simulink model "MATE_IEEE123Node"  (R2024b)
settings: Solver=FixedStepDiscrete  StartTime=0.0  StopTime=1  FixedStep=Ts  RelTol=1e-3
PostLoadFcn:
  | Ts=50e-6;init_IEEE123Node;
InitFcn:
  | Ts=50e-6;init_IEEE123Node;
undefined symbols (not defined in the file): ft2km, loadcoeff, MATE, MATERT, Pa1, Pa13, Pa14, Pa17, Pa18, Pa22, Pa24, Pa25, Pa29, Pa31, Pa32, Pa33, Pa34, Pa35, Pa37, Pa38, Pa39, Pa44, Pa46, Pa48, Pa50, Pa51, Pa52, Pa53, Pa57, Pa59, Pa6, Pa61, Pa67, Pa7, Pa70, Pa73, Pa8, Pa81, Pa82, Pa83, Pa84, Pa85, Pa9, Pb10, Pb15, Pb2, Pb30, Pb33, Pb34, Pb35, Pb41, Pb42, Pb43, Pb47, Pb48, Pb57, Pb58, Pb60, Pb65, Pb66 ... (+124)
libraries: simetranss x259, ee_lib x93, fl_lib x67, nesl_utility x67, simetran x2
(part 2 of 4)

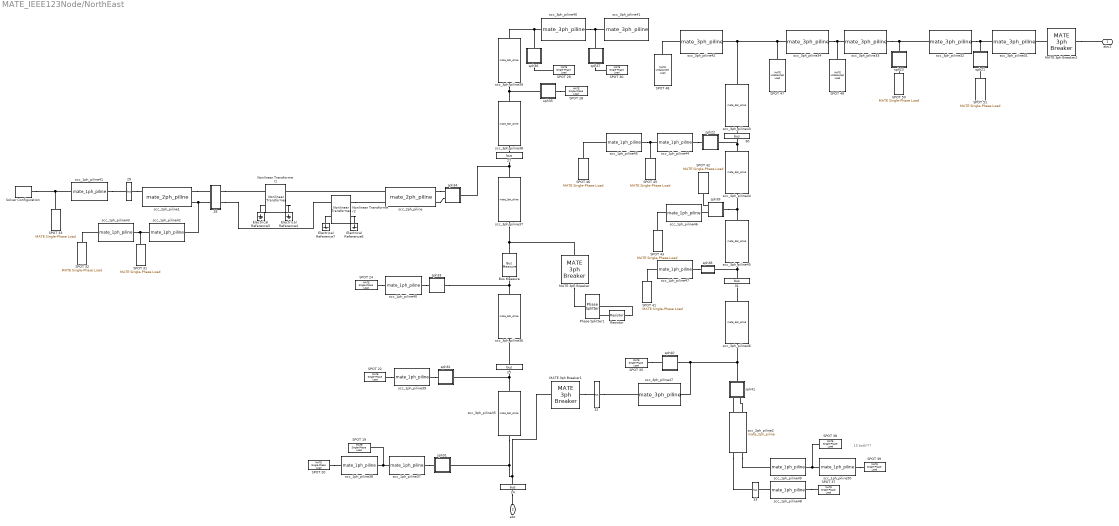
== system MATE_IEEE123Node/NorthEast ==
  note: 15 both???
  24 : simetranss/Measure/bus  bn=18
      settings: AttributesFormatString=Bus %<bn>
  25 : simetranss/Measure/bus  bn=21
      settings: AttributesFormatString=Bus %<bn>
  27 : simetranss/Measure/bus  bn=25
      settings: AttributesFormatString=Bus %<bn>
  28 : Subsystem  AncestorBlock=simetran/5  mask(Simscape Electrical Bus Numbering){bn=26}
      mask prompts: bn "Bus number"
      mask help: This block is a simple passthrough
      settings: AttributesFormatString=Bus %<bn>
  29 : simetranss/Measure/bus  bn=27
      settings: AttributesFormatString=Bus %<bn>
  30 : simetranss/Measure/bus  bn=44
      settings: AttributesFormatString=Bus %<bn>
  31 : simetranss/Measure/bus  bn=40
      settings: AttributesFormatString=Bus %<bn>
  32 : simetranss/Measure/bus  bn=135
      settings: AttributesFormatString=Bus %<bn>
  33 : simetranss/Measure/bus  bn=36
      settings: AttributesFormatString=Bus %<bn>
  Bus Measure : simetranss/Measure/Bus Measure  VoltageMeasurement=phase-to-ground  SetLabelV=on  LabelV=Vabc_B1ssc  Vpu=off  VpuLL=off  CurrentMeasurement=yes  SetLabelI=on  LabelI=Iabc_B1ssc  Ipu=off  Pbase=100e6  Vbase=500e3  bnumber=23  dis=off
  Electrical Reference{4..7} (4 alike) : fl_lib/Electrical/Electrical Elements/Electrical Reference
  MATE 3ph Breaker : simetranss/Switches/MATE 3ph Breaker  InitialState=open  SwitchA=off  SwitchB=on  SwitchC=on  SwitchTimes=[0.5 0.5+3/60]  External=off  BreakerResistance=0.01  Roff=1e6  SnubberResistance=1e6  SnubberCapacitance=inf
  MATE 3ph Breaker1 : simetranss/Switches/MATE 3ph Breaker  InitialState=closed  SwitchA=off  SwitchB=off  SwitchC=off  SwitchTimes="[1/60  5/60]"  External=off  BreakerResistance=0.01  Roff=1e6  SnubberResistance=1e6  SnubberCapacitance=inf
  MATE 3ph Breaker2 : simetranss/Switches/MATE 3ph Breaker  InitialState=closed  SwitchA=off  SwitchB=off  SwitchC=off  SwitchTimes="[1/60  5/60]"  External=off  BreakerResistance=0.01  Roff=1e6  SnubberResistance=1e6  SnubberCapacitance=inf
  Nonlinear Transformer1 : ee_lib/Passive/Transformers/Nonlinear Transformer  Nw=1  Nw2=1  winding_param_option=2  Req=0.01 Ohm  Leq=0.0001 H  R_1=0.087552 Ohm  L_1=0.011426 H  R_2=0.27563 Ohm  L_2=0.035971 H  averaging_period=0 s  R_m=50000 Ohm  parameterization_option=1  H_data=[0, 200, 400, 600, 800, 1000] A/m  B_data=[0, .81, 1.25, 1.42, 1.48, 1.49] T  length_effective=0.2 m  area_effective=2e-4 m^2  L=1 H  L_sat=1e-2 H  current_data=[0, .4, .8, 1.2, 1.6, 2] A  magnetic_flux_data=[0, .161, .25, .284, .295, .299] .* 1e-3 Wb  magnetic_flux_sat=1.6e-04 Wb  dBdH0=0.005 T*m/A  B1=1.49 T  H1=1000 A/m  c=0.1  K=200 A/m  alpha=1e-4  interpolation_option=1  Leq_i0=0 A  L1_i0=0 A  L2_i0=0 A  x0_option=1  i_L0=0 A  phi0=0 Wb  B0=0 T  H0=0 A/m  Leq_g=1e-9 1/Ohm  L1_g=1e-9 1/Ohm  L2_g=1e-9 1/Ohm
      settings: InternalSimscapePortConfiguration="{\"Bottom\":[],\"Left\":[{\"id\":\"p1\",\"label\":\"1+\",\"type\":\"foundation.electrical.electrical\"},{\"id\":\"n1\",\"label\":\"1-\",\"type\":\"foundation.electrical.electrical\"}],\"Right\":[{\"id\":\"p2\",\"label\":\"2+\",\"type\":\"foundation.electrical.electrical\"},{\"id\":\"n2\",\"label\":\"2-\",\"type\":\"foundation.electrical.electrical\"}],\"Top\":[]}"
  Nonlinear Transformer2 : ee_lib/Passive/Transformers/Nonlinear Transformer  Nw=1  Nw2=1  winding_param_option=2  Req=0.01 Ohm  Leq=0.0001 H  R_1=0.087552 Ohm  L_1=0.011426 H  R_2=0.27563 Ohm  L_2=0.035971 H  averaging_period=0 s  R_m=50000 Ohm  parameterization_option=1  H_data=[0, 200, 400, 600, 800, 1000] A/m  B_data=[0, .81, 1.25, 1.42, 1.48, 1.49] T  length_effective=0.2 m  area_effective=2e-4 m^2  L=1 H  L_sat=1e-2 H  current_data=[0, .4, .8, 1.2, 1.6, 2] A  magnetic_flux_data=[0, .161, .25, .284, .295, .299] .* 1e-3 Wb  magnetic_flux_sat=1.6e-04 Wb  dBdH0=0.005 T*m/A  B1=1.49 T  H1=1000 A/m  c=0.1  K=200 A/m  alpha=1e-4  interpolation_option=1  Leq_i0=0 A  L1_i0=0 A  L2_i0=0 A  x0_option=1  i_L0=0 A  phi0=0 Wb  B0=0 T  H0=0 A/m  Leq_g=1e-9 1/Ohm  L1_g=1e-9 1/Ohm  L2_g=1e-9 1/Ohm
      settings: InternalSimscapePortConfiguration="{\"Bottom\":[],\"Left\":[{\"id\":\"p1\",\"label\":\"1+\",\"type\":\"foundation.electrical.electrical\"},{\"id\":\"n1\",\"label\":\"1-\",\"type\":\"foundation.electrical.electrical\"}],\"Right\":[{\"id\":\"p2\",\"label\":\"2+\",\"type\":\"foundation.electrical.electrical\"},{\"id\":\"n2\",\"label\":\"2-\",\"type\":\"foundation.electrical.electrical\"}],\"Top\":[]}"
  Phase Splitter1 : ee_lib/Connectors & References/Phase Splitter
  Resistor : ee_lib/Passive/Resistor  R=0.001 Ohm  enable_R_tol=ee.enum.toleranceApplication.none  R_tol=5  tol_distribution=ee.enum.toleranceDistribution.uniform  nSigma=4  enable_operating_limits=ee.enum.enable.no  operating_limit_action=ee.enum.passive.reportOpLim.warn  power_rating=1 W  max_working_voltage=100 V  noise_mode=ee.enum.sources.noise.Disabled  Tdevice=25 degC  sample_time=1e-3 s  repeatability=ee.enum.ic.repeatability.notRepeatable  user_seed=0  auto_seed=2080827355  fault_action=simscape.enum.assert.action.none  t_fault=1 s  power_derating_T1=70 degC  power_derating_T2=155 degC  operating_temperature_range_vec=[-50, 150] degC  alpha=3.93e-3 1/K  Tmeas=25 degC  thermal_mass=100 J/K  temperature_specify=off  temperature_priority=High  temperature=298.15 K  temperature_nominal_specify=off  temperature_nominal_value=1  temperature_nominal_unit=K
  SPOT 19 : simetranss/Passive/MATE Single-Phase Load  Vabc=VsubL/sqrt(3)  Fn=60  typ=Series RL  Pabc=Pa13*loadcoeff  QLabc=Qa13*loadcoeff  QCabc="[190  ]*1e3"
  SPOT 20 : simetranss/Passive/MATE Single-Phase Load  Vabc=VsubL/sqrt(3)  Fn=60  typ=Series RL  Pabc=Pa14*loadcoeff  QLabc=Qa14*loadcoeff  QCabc="[190  ]*1e3"
  SPOT 22 : simetranss/Passive/MATE Single-Phase Load  Vabc=VsubL/sqrt(3)  Fn=60  typ=Series RL  Pabc=Pb15*loadcoeff  QLabc=Qb15*loadcoeff  QCabc="[190  ]*1e3"
  SPOT 24 : simetranss/Passive/MATE Single-Phase Load  Vabc=VsubL/sqrt(3)  Fn=60  typ=Series RL  Pabc=Pc16*loadcoeff  QLabc=Qc16*loadcoeff  QCabc="[190  ]*1e3"
  SPOT 28 : simetranss/Passive/MATE Single-Phase Load  Vabc=VsubL/sqrt(3)  Fn=60  typ=Series RL  Pabc=Pa17*loadcoeff  QLabc=Qa17*loadcoeff  QCabc="[190  ]*1e3"
  SPOT 29 : simetranss/Passive/MATE Single-Phase Load  Vabc=VsubL/sqrt(3)  Fn=60  typ=Series RL  Pabc=Pa18*loadcoeff  QLabc=Qa18*loadcoeff  QCabc="[190  ]*1e3"
  SPOT 30 : simetranss/Passive/MATE Single-Phase Load  Vabc=VsubL/sqrt(3)  Fn=60  typ=Series RL  Pabc=Pc19*loadcoeff  QLabc=Qc19*loadcoeff  QCabc="[190  ]*1e3"
  SPOT 31 : simetranss/Passive/MATE Single-Phase Load  Vabc=VsubL/sqrt(3)  Fn=60  typ=Series RL  Pabc=Pc20*loadcoeff  QLabc=Qc20*loadcoeff  QCabc="[190  ]*1e3"
  SPOT 32 : simetranss/Passive/MATE Single-Phase Load  Vabc=VsubL/sqrt(3)  Fn=60  typ=Series RL  Pabc=Pc21*loadcoeff  QLabc=Qc21*loadcoeff  QCabc="[190  ]*1e3"
  SPOT 33 : simetranss/Passive/MATE Single-Phase Load  Vabc=VsubL/sqrt(3)  Fn=60  typ=Series RL  Pabc=Pa22*loadcoeff  QLabc=Qa22*loadcoeff  QCabc="[190  ]*1e3"
  SPOT 35 : simetranss/Passive/MATE Single-Phase Load  Vabc=VsubL/sqrt(3)  Fn=60  typ=Series RL  Pabc=Pa24*loadcoeff  QLabc=Qa24*loadcoeff  QCabc="[190  ]*1e3"
  SPOT 37 : simetranss/Passive/MATE Single-Phase Load  Vabc=VsubL/sqrt(3)  Fn=60  typ=Series RL  Pabc=Pa25*loadcoeff  QLabc=Qa25*loadcoeff  QCabc="[190  ]*1e3"
  SPOT 38 : simetranss/Passive/MATE Single-Phase Load  Vabc=VsubL/sqrt(3)  Fn=60  typ=Series RL  Pabc=Pb15*loadcoeff  QLabc=Qb15*loadcoeff  QCabc="[190  ]*1e3"
  SPOT 39 : simetranss/Passive/MATE Single-Phase Load  Vabc=VsubL/sqrt(3)  Fn=60  typ=Series RL  Pabc=Pb15*loadcoeff  QLabc=Qb15*loadcoeff  QCabc="[190  ]*1e3"
  SPOT 41 : simetranss/Passive/MATE Single-Phase Load  Vabc=VsubL/sqrt(3)  Fn=60  typ=Series RL  Pabc=Pc28*loadcoeff  QLabc=Qc28*loadcoeff  QCabc="[190  ]*1e3"
  SPOT 42 : simetranss/Passive/MATE Single-Phase Load  Vabc=VsubL/sqrt(3)  Fn=60  typ=Series RL  Pabc=Pa29*loadcoeff  QLabc=Qa29*loadcoeff  QCabc="[190  ]*1e3"
  SPOT 43 : simetranss/Passive/MATE Single-Phase Load  Vabc=VsubL/sqrt(3)  Fn=60  typ=Series RL  Pabc=Pb30*loadcoeff  QLabc=Qb30*loadcoeff  QCabc="[190  ]*1e3"
  SPOT 45 : simetranss/Passive/MATE Single-Phase Load  Vabc=VsubL/sqrt(3)  Fn=60  typ=Series RL  Pabc=Pa31*loadcoeff  QLabc=Qa31*loadcoeff  QCabc="[190  ]*1e3"
  SPOT 46 : simetranss/Passive/MATE Single-Phase Load  Vabc=VsubL/sqrt(3)  Fn=60  typ=Series RL  Pabc=Pa32*loadcoeff  QLabc=Qa32*loadcoeff  QCabc="[190  ]*1e3"
  SPOT 47 : simetranss/Passive/MATE Unbalanced Load  Vabc=[ 0.993926 1.02168 0.995885]*277.128  Fn=60  typ=Series RL  Pabc=[Pa33*loadcoeff Pb33*loadcoeff Pc33*loadcoeff]  QLabc=[Qa33*loadcoeff Qb33*loadcoeff Qc33*loadcoeff]  QCabc="[190  60  212]*1e3"
  SPOT 48 : simetranss/Passive/MATE Unbalanced Load  Vabc=[ 0.993926 1.02168 0.995885]*277.128  Fn=60  typ=Series RL  Pabc=[Pa34*loadcoeff Pb34*loadcoeff Pc34*loadcoeff]  QLabc=[Qa34*loadcoeff Qb34*loadcoeff Qc34*loadcoeff]  QCabc="[190  60  212]*1e3"
  SPOT 49 : simetranss/Passive/MATE Unbalanced Load  Vabc=[ 0.993926 1.02168 0.995885]*277.128  Fn=60  typ=Series RL  Pabc=[Pa35*loadcoeff Pb35*loadcoeff Pc35*loadcoeff]  QLabc=[Qa35*loadcoeff Qb35*loadcoeff Qc35*loadcoeff]  QCabc="[190  60  212]*1e3"
  SPOT 50 : simetranss/Passive/MATE Single-Phase Load  Vabc=VsubL/sqrt(3)  Fn=60  typ=Series RL  Pabc=Pc36*loadcoeff  QLabc=Qc36*loadcoeff  QCabc="[190  ]*1e3"
  SPOT 51 : simetranss/Passive/MATE Single-Phase Load  Vabc=VsubL/sqrt(3)  Fn=60  typ=Series RL  Pabc=Pa37*loadcoeff  QLabc=Qa37*loadcoeff  QCabc="[190  ]*1e3"
  Solver Configuration : nesl_utility/Solver Configuration  PhysicalDomain=network_engine_domain  SubClassName=solver  LeftPortType=input  RightPortType=generic  Tones=[]  Harmonics=[]  SimulateNoise=off  Profile=off  UseLocalSampling=off  EnableSwitchedLinearOptims=on  FrequencyDomain=off  UseCCode=off  RelTol=0.001  AbsTol=0.001  MinStep=1e-09  ToWorkspace=off  RevertToSquareIcSolve=off  NumHomotopyIterations=100  PhasorMode=off  PhasorModeNumHarmonics=1  ConsistencySolver=NEWTON_XTOL_AFTER_FTOL  IndexReductionMethod=None  DoDC=off  ResidualTolerance=1e-09  ConsistencyTolSource=GLOBAL  ConsistencyAbsTol=0.001  ConsistencyRelTol=0.001  ConsistencyTolFactor=0.1  UseLocalSolver=on  LocalSolverChoice=NE_PARTITIONING_ADVANCER  ResolveIndetEquations=off  FunctionEvalNumThread=1  LocalSolverSampleTime=Ts  DoFixedCost=on  MaxNonlinIter=1  MaxModeIter=2  ComputeImpulses=off  ImpulseIterations=2  LinearAlgebra=auto  LinearAlgebraNumThread=0  EquationFormulation=NE_TIME_EF  DelaysMemoryBudget=1024  AutomaticFiltering=on  FilteringTimeConstant=0.001  PartitionStorageMethod=AS_NEEDED  PartitionMemoryBudget=1024  PartitionMethod=ROBUST  MultibodyUseLocalSolver=off  MultibodyLocalSolverChoice=ODE1  MultibodyLocalSolverSampleTime=0.001
  scc_1ph_piline37 : simetranss/Lines/mate_1ph_piline  FF=60  conf=config 9  lenfeet=250  dmi=off  RR1=0.8  LL1=0.002  CC1=7e-9  lenkm=1
  scc_1ph_piline38 : simetranss/Lines/mate_1ph_piline  FF=60  conf=config 9  lenfeet=325  dmi=off  RR1=0.8  LL1=0.002  CC1=7e-9  lenkm=1
  scc_1ph_piline39 : simetranss/Lines/mate_1ph_piline  FF=60  conf=config 10  lenfeet=525  dmi=off  RR1=0.8  LL1=0.002  CC1=7e-9  lenkm=1
  scc_1ph_piline40 : simetranss/Lines/mate_1ph_piline  FF=60  conf=config 11  lenfeet=550  dmi=off  RR1=0.8  LL1=0.002  CC1=7e-9  lenkm=1
  scc_1ph_piline41 : simetranss/Lines/mate_1ph_piline  FF=60  conf=config 9  lenfeet=500  dmi=off  RR1=0.8  LL1=0.002  CC1=7e-9  lenkm=1
  scc_1ph_piline42 : simetranss/Lines/mate_1ph_piline  FF=60  conf=config 11  lenfeet=225  dmi=off  RR1=0.8  LL1=0.002  CC1=7e-9  lenkm=1
  scc_1ph_piline43 : simetranss/Lines/mate_1ph_piline  FF=60  conf=config 11  lenfeet=300  dmi=off  RR1=0.8  LL1=0.002  CC1=7e-9  lenkm=1
  scc_1ph_piline44 : simetranss/Lines/mate_1ph_piline  FF=60  conf=config 9  lenfeet=200  dmi=off  RR1=0.8  LL1=0.002  CC1=7e-9  lenkm=1
  scc_1ph_piline45 : simetranss/Lines/mate_1ph_piline  FF=60  conf=config 9  lenfeet=300  dmi=off  RR1=0.8  LL1=0.002  CC1=7e-9  lenkm=1
  scc_1ph_piline46 : simetranss/Lines/mate_1ph_piline  FF=60  conf=config 10  lenfeet=500  dmi=off  RR1=0.8  LL1=0.002  CC1=7e-9  lenkm=1
  scc_1ph_piline47 : simetranss/Lines/mate_1ph_piline  FF=60  conf=config 11  lenfeet=325  dmi=off  RR1=0.8  LL1=0.002  CC1=7e-9  lenkm=1
  scc_1ph_piline48 : simetranss/Lines/mate_1ph_piline  FF=60  conf=config 9  lenfeet=300  dmi=off  RR1=0.8  LL1=0.002  CC1=7e-9  lenkm=1
  scc_1ph_piline49 : simetranss/Lines/mate_1ph_piline  FF=60  conf=config 10  lenfeet=250  dmi=off  RR1=0.8  LL1=0.002  CC1=7e-9  lenkm=1
  scc_1ph_piline50 : simetranss/Lines/mate_1ph_piline  FF=60  conf=config 10  lenfeet=325  dmi=off  RR1=0.8  LL1=0.002  CC1=7e-9  lenkm=1
  scc_2ph_piline : simetranss/Lines/mate_2ph_piline  FF=60  conf=config 7  lenfeet=350  dmi=off  RR22=[1 0; 0 1]  LL22=[1 0; 0 1]  CC22=[1 0; 0 1]  lenkm=1
  scc_2ph_piline1 : simetranss/Lines/mate_2ph_piline  FF=60  conf=config 7  lenfeet=275  dmi=off  RR22=[1 0; 0 1]  LL22=[1 0; 0 1]  CC22=[1 0; 0 1]  lenkm=1
  scc_2ph_piline2 : simetranss/Lines/mate_2ph_piline  FF=60  conf=config 8  lenfeet=650  dmi=off  RR22=[1 0; 0 1]  LL22=[1 0; 0 1]  CC22=[1 0; 0 1]  lenkm=1
  scc_3ph_piline31 : simetranss/Lines/mate_3ph_piline  FF=60  conf=config 5  lenfeet=500  dmi=off  RR33=[1 0 0;0 1 0; 0 0 1]  LL33=[1 0 0;0 1 0; 0 0 1]  CC33=[1 0 0;0 1 0; 0 0 1]  lenkm=1
  scc_3ph_piline32 : simetranss/Lines/mate_3ph_piline  FF=60  conf=config 4  lenfeet=250  dmi=off  RR33=[1 0 0;0 1 0; 0 0 1]  LL33=[1 0 0;0 1 0; 0 0 1]  CC33=[1 0 0;0 1 0; 0 0 1]  lenkm=1
  scc_3ph_piline33 : simetranss/Lines/mate_3ph_piline  FF=60  conf=config 4  lenfeet=250  dmi=off  RR33=[1 0 0;0 1 0; 0 0 1]  LL33=[1 0 0;0 1 0; 0 0 1]  CC33=[1 0 0;0 1 0; 0 0 1]  lenkm=1
  scc_3ph_piline34 : simetranss/Lines/mate_3ph_piline  FF=60  conf=config 4  lenfeet=250  dmi=off  RR33=[1 0 0;0 1 0; 0 0 1]  LL33=[1 0 0;0 1 0; 0 0 1]  CC33=[1 0 0;0 1 0; 0 0 1]  lenkm=1
  scc_3ph_piline35 : simetranss/Lines/mate_3ph_piline  FF=60  conf=config 2  lenfeet=300  dmi=off  RR33=[1 0 0;0 1 0; 0 0 1]  LL33=[1 0 0;0 1 0; 0 0 1]  CC33=[1 0 0;0 1 0; 0 0 1]  lenkm=1
  scc_3ph_piline36 : simetranss/Lines/mate_3ph_piline  FF=60  conf=config 2  lenfeet=250  dmi=off  RR33=[1 0 0;0 1 0; 0 0 1]  LL33=[1 0 0;0 1 0; 0 0 1]  CC33=[1 0 0;0 1 0; 0 0 1]  lenkm=1
  scc_3ph_piline37 : simetranss/Lines/mate_3ph_piline  FF=60  conf=config 2  lenfeet=275  dmi=off  RR33=[1 0 0;0 1 0; 0 0 1]  LL33=[1 0 0;0 1 0; 0 0 1]  CC33=[1 0 0;0 1 0; 0 0 1]  lenkm=1
  scc_3ph_piline38 : simetranss/Lines/mate_3ph_piline  FF=60  conf=config 2  lenfeet=200  dmi=off  RR33=[1 0 0;0 1 0; 0 0 1]  LL33=[1 0 0;0 1 0; 0 0 1]  CC33=[1 0 0;0 1 0; 0 0 1]  lenkm=1
  scc_3ph_piline39 : simetranss/Lines/mate_3ph_piline  FF=60  conf=config 2  lenfeet=300  dmi=off  RR33=[1 0 0;0 1 0; 0 0 1]  LL33=[1 0 0;0 1 0; 0 0 1]  CC33=[1 0 0;0 1 0; 0 0 1]  lenkm=1
  scc_3ph_piline40 : simetranss/Lines/mate_3ph_piline  FF=60  conf=config 2  lenfeet=350  dmi=off  RR33=[1 0 0;0 1 0; 0 0 1]  LL33=[1 0 0;0 1 0; 0 0 1]  CC33=[1 0 0;0 1 0; 0 0 1]  lenkm=1
  scc_3ph_piline41 : simetranss/Lines/mate_3ph_piline  FF=60  conf=config 2  lenfeet=200  dmi=off  RR33=[1 0 0;0 1 0; 0 0 1]  LL33=[1 0 0;0 1 0; 0 0 1]  CC33=[1 0 0;0 1 0; 0 0 1]  lenkm=1
  scc_3ph_piline42 : simetranss/Lines/mate_3ph_piline  FF=60  conf=config 4  lenfeet=150  dmi=off  RR33=[1 0 0;0 1 0; 0 0 1]  LL33=[1 0 0;0 1 0; 0 0 1]  CC33=[1 0 0;0 1 0; 0 0 1]  lenkm=1
  scc_3ph_piline43 : simetranss/Lines/mate_3ph_piline  FF=60  conf=config 1  lenfeet=250  dmi=off  RR33=[1 0 0;0 1 0; 0 0 1]  LL33=[1 0 0;0 1 0; 0 0 1]  CC33=[1 0 0;0 1 0; 0 0 1]  lenkm=1
  scc_3ph_piline44 : simetranss/Lines/mate_3ph_piline  FF=60  conf=config 1  lenfeet=200  dmi=off  RR33=[1 0 0;0 1 0; 0 0 1]  LL33=[1 0 0;0 1 0; 0 0 1]  CC33=[1 0 0;0 1 0; 0 0 1]  lenkm=1
  scc_3ph_piline45 : simetranss/Lines/mate_3ph_piline  FF=60  conf=config 1  lenfeet=250  dmi=off  RR33=[1 0 0;0 1 0; 0 0 1]  LL33=[1 0 0;0 1 0; 0 0 1]  CC33=[1 0 0;0 1 0; 0 0 1]  lenkm=1
  scc_3ph_piline46 : simetranss/Lines/mate_3ph_piline  FF=60  conf=config 1  lenfeet=250  dmi=off  RR33=[1 0 0;0 1 0; 0 0 1]  LL33=[1 0 0;0 1 0; 0 0 1]  CC33=[1 0 0;0 1 0; 0 0 1]  lenkm=1
  scc_3ph_piline47 : simetranss/Lines/mate_3ph_piline  FF=60  conf=config 4  lenfeet=375  dmi=off  RR33=[1 0 0;0 1 0; 0 0 1]  LL33=[1 0 0;0 1 0; 0 0 1]  CC33=[1 0 0;0 1 0; 0 0 1]  lenkm=1
  sph21 : Subsystem
  sph22 : Subsystem
  sph23 : Subsystem
  sph31 : Subsystem
  sph32 : Subsystem
  sph33 : Subsystem
  sph34 : Subsystem
  sph35 : Subsystem
  sph36 : Subsystem
  sph37 : Subsystem
  sph38 : Subsystem
  sph39 : Subsystem
  sph40 : Subsystem
  sph41 : Subsystem
  abc2 : PMIOPort  Side=Right
  abc : PMIOPort  Port=2  Side=Left
  connections:
  scc_3ph_piline34/LConn1 -- SPOT 47/LConn1 -- scc_3ph_piline42/RConn1 -- scc_3ph_piline43/LConn1
  27/LConn1 -- scc_3ph_piline37/LConn1 -- sph34/LConn1
  scc_3ph_piline32/RConn1 -- scc_3ph_piline31/LConn1 -- sph21/LConn1
  scc_3ph_piline46/RConn1 -- scc_3ph_piline47/LConn1 -- sph40/LConn1 -- sph41/LConn1
  scc_3ph_piline34/RConn1 -- scc_3ph_piline33/LConn1 -- SPOT 49/LConn1
  scc_3ph_piline39/LConn1 -- sph36/LConn1 -- scc_3ph_piline40/RConn1
  scc_1ph_piline46/RConn1 -- SPOT 43/LConn1
  scc_1ph_piline43/LConn1 -- SPOT 32/LConn1
  scc_3ph_piline37/RConn1 -- Bus Measure/LConn1 -- MATE 3ph Breaker/LConn1
  scc_2ph_piline2/RConn2 -- scc_1ph_piline49/RConn1
  SPOT 41/LConn1 -- scc_1ph_piline47/RConn1
  scc_1ph_piline39/LConn1 -- sph32/RConn1
  30/RConn1 -- scc_3ph_piline43/RConn1
  28/RConn2 -- Nonlinear Transformer2/LConn1
  scc_3ph_piline35/LConn1 -- 25/LConn1 -- sph32/LConn1
  scc_2ph_piline2/LConn1 -- sph41/RConn1
  sph37/RConn1 -- SPOT 30/LConn1
  sph39/RConn2 -- scc_1ph_piline46/LConn1
  31/RConn1 -- scc_3ph_piline45/RConn1 -- sph38/LConn1
  scc_3ph_piline44/LConn1 -- sph22/LConn1 -- 30/LConn1
  scc_3ph_piline33/RConn1 -- scc_3ph_piline32/LConn1 -- sph23/LConn1
  SPOT 51/LConn1 -- sph21/RConn1
  scc_1ph_piline48/LConn1 -- SPOT 37/LConn1
  scc_3ph_piline39/RConn1 -- scc_3ph_piline38/LConn1 -- sph35/LConn1
  MATE 3ph Breaker1/LConn1 -- 32/LConn1
  25/RConn1 -- scc_3ph_piline36/RConn1
  scc_3ph_piline46/LConn1 -- 31/LConn1
  Nonlinear Transformer2/LConn2 -- Electrical Reference7/LConn1
  SPOT 22/LConn1 -- scc_1ph_piline39/RConn1
  scc_1ph_piline49/LConn1 -- SPOT 38/LConn1 -- scc_1ph_piline50/RConn1
  sph39/RConn1 -- SPOT 42/LConn1
  scc_2ph_piline1/RConn2 -- scc_1ph_piline42/RConn1 -- 28/LConn2
  28/RConn1 -- Nonlinear Transformer1/LConn1
  scc_2ph_piline2/RConn1 -- 33/LConn1
  sph35/RConn1 -- SPOT 28/LConn1
  Nonlinear Transformer1/LConn2 -- Electrical Reference5/LConn1
  scc_1ph_piline40/LConn1 -- sph33/RConn1
  scc_1ph_piline44/LConn1 -- sph22/RConn1
  scc_1ph_piline47/LConn1 -- sph38/RConn1
  SPOT 20/LConn1 -- scc_1ph_piline38/RConn1
  scc_1ph_piline41/RConn1 -- 29/RConn1
  scc_1ph_piline37/LConn1 -- sph31/RConn1
  MATE 3ph Breaker2/RConn1 -- abc2/RConn1
  scc_1ph_piline38/LConn1 -- SPOT 19/LConn1 -- scc_1ph_piline37/RConn1
  SPOT 50/LConn1 -- sph23/RConn1
  32/RConn1 -- scc_3ph_piline47/RConn1
  MATE 3ph Breaker2/LConn1 -- scc_3ph_piline31/RConn1
  scc_3ph_piline40/LConn1 -- sph37/LConn1 -- scc_3ph_piline41/RConn1
  scc_2ph_piline2/LConn2 -- sph41/RConn2
  scc_1ph_piline48/RConn1 -- 33/RConn1
  scc_2ph_piline1/RConn1 -- 28/LConn1
  scc_3ph_piline44/RConn1 -- sph39/LConn1 -- scc_3ph_piline45/LConn1
  scc_1ph_piline43/RConn1 -- SPOT 31/LConn1 -- scc_1ph_piline42/LConn1
  SPOT 46/LConn1 -- scc_1ph_piline45/RConn1
  SPOT 24/LConn1 -- scc_1ph_piline40/RConn1
  scc_3ph_piline35/RConn1 -- sph31/LConn1 -- MATE 3ph Breaker1/RConn1 -- 24/RConn1
  Nonlinear Transformer2/RConn2 -- Electrical Reference6/LConn1
  sph36/RConn1 -- SPOT 29/LConn1
  scc_3ph_piline38/RConn1 -- 27/RConn1
  scc_1ph_piline45/LConn1 -- SPOT 45/LConn1 -- scc_1ph_piline44/RConn1
  29/LConn1 -- scc_2ph_piline1/LConn1
  scc_2ph_piline/RConn2 -- sph34/RConn2
  Nonlinear Transformer1/RConn2 -- Electrical Reference4/LConn1
  SPOT 33/LConn1 -- Solver Configuration/RConn1 -- scc_1ph_piline41/LConn1
  scc_1ph_piline50/LConn1 -- SPOT 39/LConn1
  SPOT 35/LConn1 -- sph40/RConn1
  scc_2ph_piline/LConn1 -- Nonlinear Transformer1/RConn1
  scc_2ph_piline/RConn1 -- sph34/RConn1
  Nonlinear Transformer2/RConn1 -- scc_2ph_piline/LConn2
  24/LConn1 -- abc/RConn1
  sph33/LConn1 -- Bus Measure/RConn1 -- scc_3ph_piline36/LConn1
  scc_3ph_piline42/LConn1 -- SPOT 48/LConn1
  MATE 3ph Breaker/RConn1 -- Phase Splitter1/LConn1
  Resistor/LConn1 -- Phase Splitter1/RConn3
  Resistor/RConn1 -- Phase Splitter1/RConn2

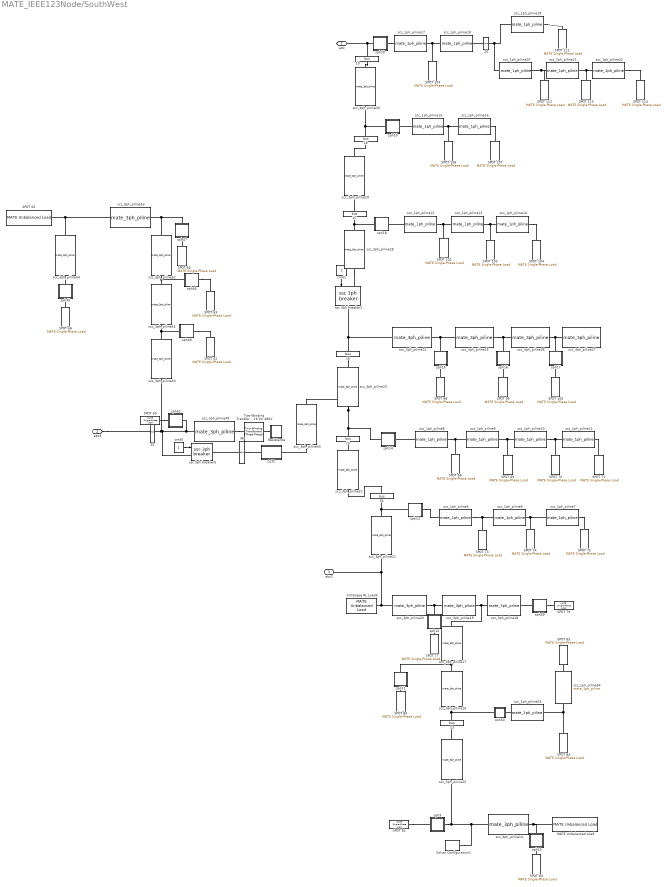
== system MATE_IEEE123Node/SouthWest ==
  13 : simetranss/Measure/bus  bn=61
      settings: AttributesFormatString=Bus %<bn>
  14 : simetranss/Measure/bus  bn=72
      settings: AttributesFormatString=Bus %<bn>
  15 : simetranss/Measure/bus  bn=67
      settings: AttributesFormatString=Bus %<bn>
  16 : simetranss/Measure/bus  bn=97
      settings: AttributesFormatString=Bus %<bn>
  17 : simetranss/Measure/bus  bn=97
      settings: AttributesFormatString=Bus %<bn>
  18 : simetranss/Measure/bus  bn=105
      settings: AttributesFormatString=Bus %<bn>
  19 : simetranss/Measure/bus  bn=108
      settings: AttributesFormatString=Bus %<bn>
  20 : simetranss/Measure/bus  bn=110
      settings: AttributesFormatString=Bus %<bn>
  35 : simetranss/Measure/bus  bn=60
      settings: AttributesFormatString=Bus %<bn>
  36 : simetranss/Measure/bus  bn=160
      settings: AttributesFormatString=Bus %<bn>
  MATE Unbalanced Load : simetranss/Passive/MATE Unbalanced Load  Vabc=[VsubL/sqrt(3) VsubL/sqrt(3) VsubL/sqrt(3)]  Fn=60  typ=Capacitance  Pabc=[160 120 120]*1e3  QLabc=[110 90 90]*1e3  QCabc=[200 200 200]*1e3
  OLTC : Subsystem
  Resistance : Subsystem  mask{R=[1e5 1e5 1e5]}
      mask prompts: R "Resistances phase a b c (Ohms)"
  SPOT 100 : simetranss/Passive/MATE Single-Phase Load  Vabc=VsubL/sqrt(3)  Fn=60  typ=Series RL  Pabc=Pc75*loadcoeff  QLabc=Qc75*loadcoeff  QCabc="[190  ]*1e3"
  SPOT 102 : simetranss/Passive/MATE Single-Phase Load  Vabc=VsubL/sqrt(3)  Fn=60  typ=Series RL  Pabc=Pc76*loadcoeff  QLabc=Qc76*loadcoeff  QCabc="[190  ]*1e3"
  SPOT 103 : simetranss/Passive/MATE Single-Phase Load  Vabc=VsubL/sqrt(3)  Fn=60  typ=Series RL  Pabc=Pc77*loadcoeff  QLabc=Qc77*loadcoeff  QCabc="[190  ]*1e3"
  SPOT 104 : simetranss/Passive/MATE Single-Phase Load  Vabc=VsubL/sqrt(3)  Fn=60  typ=Series RL  Pabc=Pc78*loadcoeff  QLabc=Qc78*loadcoeff  QCabc="[190  ]*1e3"
  SPOT 106 : simetranss/Passive/MATE Single-Phase Load  Vabc=VsubL/sqrt(3)  Fn=60  typ=Series RL  Pabc=Pb79*loadcoeff  QLabc=Qb79*loadcoeff  QCabc="[190  ]*1e3"
  SPOT 107 : simetranss/Passive/MATE Single-Phase Load  Vabc=VsubL/sqrt(3)  Fn=60  typ=Series RL  Pabc=Pb80*loadcoeff  QLabc=Qb80*loadcoeff  QCabc="[190  ]*1e3"
  SPOT 109 : simetranss/Passive/MATE Single-Phase Load  Vabc=VsubL/sqrt(3)  Fn=60  typ=Series RL  Pabc=Pa81*loadcoeff  QLabc=Qa81*loadcoeff  QCabc="[190  ]*1e3"
  SPOT 111 : simetranss/Passive/MATE Single-Phase Load  Vabc=VsubL/sqrt(3)  Fn=60  typ=Series RL  Pabc=Pa82*loadcoeff  QLabc=Qa82*loadcoeff  QCabc="[190  ]*1e3"
  SPOT 112 : simetranss/Passive/MATE Single-Phase Load  Vabc=VsubL/sqrt(3)  Fn=60  typ=Series RL  Pabc=Pa83*loadcoeff  QLabc=Qa83*loadcoeff  QCabc="[190  ]*1e3"
  SPOT 113 : simetranss/Passive/MATE Single-Phase Load  Vabc=VsubL/sqrt(3)  Fn=60  typ=Series RL  Pabc=Pa84*loadcoeff  QLabc=Qa84*loadcoeff  QCabc="[190  ]*1e3"
  SPOT 114 : simetranss/Passive/MATE Single-Phase Load  Vabc=VsubL/sqrt(3)  Fn=60  typ=Series RL  Pabc=Pa85*loadcoeff  QLabc=Qa85*loadcoeff  QCabc="[190  ]*1e3"
  SPOT 60 : simetranss/Passive/MATE Single-Phase Load  Vabc=VsubL/sqrt(3)  Fn=60  typ=Series RL  Pabc=Pa44*loadcoeff  QLabc=Qa44*loadcoeff  QCabc="[190  ]*1e3"
  SPOT 62 : simetranss/Passive/MATE Single-Phase Load  Vabc=VsubL/sqrt(3)  Fn=60  typ=Series RL  Pabc=Pc45*loadcoeff  QLabc=Qc45*loadcoeff  QCabc="[190  ]*1e3"
  SPOT 63 : simetranss/Passive/MATE Single-Phase Load  Vabc=VsubL/sqrt(3)  Fn=60  typ=Series RL  Pabc=Pa46*loadcoeff  QLabc=Qa46*loadcoeff  QCabc="[190  ]*1e3"
  SPOT 64 : simetranss/Passive/MATE Single-Phase Load  Vabc=VsubL/sqrt(3)  Fn=60  typ=Series RL  Pabc=Pb47*loadcoeff  QLabc=Pb47*loadcoeff  QCabc="[190  ]*1e3"
  SPOT 65 : simetranss/Passive/MATE Unbalanced Load  Vabc=[VsubL/sqrt(3) VsubL/sqrt(3) VsubL/sqrt(3)]  Fn=60  typ=Series RL  Pabc=[Pa48*loadcoeff Pb48*loadcoeff Pc48*loadcoeff]  QLabc=[Qa48*loadcoeff Qb48*loadcoeff Qc48*loadcoeff]  QCabc="[190  60  212]*1e3"
  SPOT 66 : simetranss/Passive/MATE Single-Phase Load  Vabc=VsubL/sqrt(3)  Fn=60  typ=Series RL  Pabc=Pc49*loadcoeff  QLabc=Qc49*loadcoeff  QCabc="[190  ]*1e3"
  SPOT 68 : simetranss/Passive/MATE Single-Phase Load  Vabc=VsubL/sqrt(3)  Fn=60  typ=Series RL  Pabc=Pa50*loadcoeff  QLabc=Qa50*loadcoeff  QCabc="[190  ]*1e3"
  SPOT 69 : simetranss/Passive/MATE Single-Phase Load  Vabc=VsubL/sqrt(3)  Fn=60  typ=Series RL  Pabc=Pa51*loadcoeff  QLabc=Qa51*loadcoeff  QCabc="[190  ]*1e3"
  SPOT 70 : simetranss/Passive/MATE Single-Phase Load  Vabc=VsubL/sqrt(3)  Fn=60  typ=Series RL  Pabc=Pa52*loadcoeff  QLabc=Qa52*loadcoeff  QCabc="[190  ]*1e3"
  SPOT 71 : simetranss/Passive/MATE Single-Phase Load  Vabc=VsubL/sqrt(3)  Fn=60  typ=Series RL  Pabc=Pa53*loadcoeff  QLabc=Qa53*loadcoeff  QCabc="[190  ]*1e3"
  SPOT 73 : simetranss/Passive/MATE Single-Phase Load  Vabc=VsubL/sqrt(3)  Fn=60  typ=Series RL  Pabc=Pc54*loadcoeff  QLabc=Qc54*loadcoeff  QCabc="[190  ]*1e3"
  SPOT 74 : simetranss/Passive/MATE Single-Phase Load  Vabc=VsubL/sqrt(3)  Fn=60  typ=Series RL  Pabc=Pc55*loadcoeff  QLabc=Qc55*loadcoeff  QCabc="[190  ]*1e3"
  SPOT 75 : simetranss/Passive/MATE Single-Phase Load  Vabc=VsubL/sqrt(3)  Fn=60  typ=Series RL  Pabc=Pc56*loadcoeff  QLabc=Qc56*loadcoeff  QCabc="[190  ]*1e3"
  SPOT 77 : simetranss/Passive/MATE Single-Phase Load  Vabc=VsubL/sqrt(3)  Fn=60  typ=Series RL  Pabc=Pb58*loadcoeff  QLabc=Qb58*loadcoeff  QCabc="[190  ]*1e3"
  SPOT 79 : simetranss/Passive/MATE Single-Phase Load  Vabc=VsubL/sqrt(3)  Fn=60  typ=Series RL  Pabc=Pa59*loadcoeff  QLabc=Qa59*loadcoeff  QCabc="[190  ]*1e3"
  SPOT 80 : simetranss/Passive/MATE Single-Phase Load  Vabc=VsubL/sqrt(3)  Fn=60  typ=Series RL  Pabc=Pb60*loadcoeff  QLabc=Qb60*loadcoeff  QCabc="[190  ]*1e3"
  SPOT 82 : simetranss/Passive/MATE Single-Phase Load  Vabc=VsubL/sqrt(3)  Fn=60  typ=Series RL  Pabc=Pa61*loadcoeff  QLabc=Qa61*loadcoeff  QCabc="[190  ]*1e3"
  SPOT 83 : simetranss/Passive/MATE Single-Phase Load  Vabc=VsubL/sqrt(3)  Fn=60  typ=Series RL  Pabc=Pc55*loadcoeff  QLabc=Qc55*loadcoeff  QCabc="[190  ]*1e3"
  SPOT 84 : simetranss/Passive/MATE Single-Phase Load  Vabc=VsubL/sqrt(3)  Fn=60  typ=Series RL  Pabc=Pc63*loadcoeff  QLabc=Qc63*loadcoeff  QCabc="[190  ]*1e3"
  SPOT 85 : simetranss/Passive/MATE Single-Phase Load  Vabc=VsubL/sqrt(3)  Fn=60  typ=Series RL  Pabc=Pc64*loadcoeff  QLabc=Qc64*loadcoeff  QCabc="[190  ]*1e3"
  SPOT 98 : simetranss/Passive/MATE Single-Phase Load  Vabc=VsubL/sqrt(3)  Fn=60  typ=Series RL  Pabc=Pa73*loadcoeff  QLabc=Qa73*loadcoeff  QCabc="[190  ]*1e3"
  SPOT 99 : simetranss/Passive/MATE Single-Phase Load  Vabc=VsubL/sqrt(3)  Fn=60  typ=Series RL  Pabc=Pb74*loadcoeff  QLabc=Qb74*loadcoeff  QCabc="[190  ]*1e3"
  SimScape RL Load3 : simetranss/Passive/MATE Unbalanced Load  Vabc=[VsubL/sqrt(3) VsubL/sqrt(3) VsubL/sqrt(3)]  Fn=60  typ=Series RL  Pabc=[Pa57*loadcoeff Pb57*loadcoeff Pc57*loadcoeff]  QLabc=[Qa57*loadcoeff Qb57*loadcoeff Qc57*loadcoeff]  QCabc="[190  60  212]*1e3"
  Solver Configuration1 : nesl_utility/Solver Configuration  PhysicalDomain=network_engine_domain  SubClassName=solver  LeftPortType=input  RightPortType=generic  Tones=[]  Harmonics=[]  SimulateNoise=off  Profile=off  UseLocalSampling=off  EnableSwitchedLinearOptims=on  FrequencyDomain=off  UseCCode=off  RelTol=0.001  AbsTol=0.001  MinStep=1e-09  ToWorkspace=off  RevertToSquareIcSolve=off  NumHomotopyIterations=100  PhasorMode=off  PhasorModeNumHarmonics=1  ConsistencySolver=NEWTON_XTOL_AFTER_FTOL  IndexReductionMethod=None  DoDC=off  ResidualTolerance=1e-09  ConsistencyTolSource=GLOBAL  ConsistencyAbsTol=0.001  ConsistencyRelTol=0.001  ConsistencyTolFactor=0.1  UseLocalSolver=on  LocalSolverChoice=NE_PARTITIONING_ADVANCER  ResolveIndetEquations=off  FunctionEvalNumThread=1  LocalSolverSampleTime=Ts  DoFixedCost=on  MaxNonlinIter=1  MaxModeIter=2  ComputeImpulses=off  ImpulseIterations=2  LinearAlgebra=auto  LinearAlgebraNumThread=0  EquationFormulation=NE_TIME_EF  DelaysMemoryBudget=1024  AutomaticFiltering=on  FilteringTimeConstant=0.001  PartitionStorageMethod=AS_NEEDED  PartitionMemoryBudget=1024  PartitionMethod=ROBUST  MultibodyUseLocalSolver=off  MultibodyLocalSolverChoice=ODE1  MultibodyLocalSolverSampleTime=0.001
  Two-Winding Transformer 4.16 kV/ 480V : ee_lib/Passive/Transformers/Two-Winding Transformer (Three-Phase)  SRated=150e3 A*V  FRated=60 Hz  Winding1Connection=ee.enum.windingconnection.delta1  VRated1=4.16e3 V  Winding2Connection=ee.enum.windingconnection.delta1  VRated2=480 V  CoreType=ee.enum.coretype.fivelimb  pu_Rw1=0.0127  pu_Rw2=0.0127  leakage_reactance_option=ee.enum.transformer_leakage.include  pu_Xl1=0.0272/2  pu_Xl2=0.0272/2  magnetizing_resistance_option=ee.enum.transformer_magnetizingResistance.exclude  pu_Rm=1000  magnetizing_reactance_option=ee.enum.transformer_magnetizingReactance.exclude  saturation_option=ee.enum.transformer_saturation.exclude  pu_Xm=100  current_data=[0, .002, 1, 2]  magnetic_flux_data=[0, 1.2, 1.5, 1.51]  pu_X0=5000  i1_specify=off  i1_priority=None  i1=[0, 0, 0] A  i1_nominal_specify=off  i1_nominal_value=1  i1_nominal_unit=A  i2_specify=off  i2_priority=None  i2=[0, 0, 0] A  i2_nominal_specify=off  i2_nominal_value=1  i2_nominal_unit=A  phi_specify=off  phi_priority=None  phi=[0, 0, 0]  phi_nominal_specify=off  phi_nominal_value=1  phi_nominal_unit=1  power_dissipated_specify=off  power_dissipated_priority=None  power_dissipated=0 W  power_dissipated_nominal_specify=off  power_dissipated_nominal_value=1  power_dissipated_nominal_unit=W
      settings: InternalSimscapePortConfiguration="{\"Bottom\":[],\"Left\":[{\"id\":\"N1\",\"label\":\"~1\",\"type\":\"foundation.electrical.three_phase\"}],\"Right\":[{\"id\":\"N2\",\"label\":\"~2\",\"type\":\"foundation.electrical.three_phase\"}],\"Top\":[]}"
  cmd1 : Constant
  cmd5 : Constant
  scc_1ph_piline10 : simetranss/Lines/mate_1ph_piline  FF=60  conf=config 9  lenfeet=325  dmi=off  RR1=0.8  LL1=0.002  CC1=7e-9  lenkm=1
  scc_1ph_piline11 : simetranss/Lines/mate_1ph_piline  FF=60  conf=config 9  lenfeet=325  dmi=off  RR1=0.8  LL1=0.002  CC1=7e-9  lenkm=1
  scc_1ph_piline12 : simetranss/Lines/mate_1ph_piline  FF=60  conf=config 11  lenfeet=225  dmi=off  RR1=0.8  LL1=0.002  CC1=7e-9  lenkm=1
  scc_1ph_piline13 : simetranss/Lines/mate_1ph_piline  FF=60  conf=config 11  lenfeet=325  dmi=off  RR1=0.8  LL1=0.002  CC1=7e-9  lenkm=1
  scc_1ph_piline14 : simetranss/Lines/mate_1ph_piline  FF=60  conf=config 11  lenfeet=700  dmi=off  RR1=0.8  LL1=0.002  CC1=7e-9  lenkm=1
  scc_1ph_piline15 : simetranss/Lines/mate_1ph_piline  FF=60  conf=config 10  lenfeet=225  dmi=off  RR1=0.8  LL1=0.002  CC1=7e-9  lenkm=1
  scc_1ph_piline16 : simetranss/Lines/mate_1ph_piline  FF=60  conf=config 10  lenfeet=575  dmi=off  RR1=0.8  LL1=0.002  CC1=7e-9  lenkm=1
  scc_1ph_piline17 : simetranss/Lines/mate_1ph_piline  FF=60  conf=config 9  lenfeet=450  dmi=off  RR1=0.8  LL1=0.002  CC1=7e-9  lenkm=1
  scc_1ph_piline18 : simetranss/Lines/mate_1ph_piline  FF=60  conf=config 9  lenfeet=300  dmi=off  RR1=0.8  LL1=0.002  CC1=7e-9  lenkm=1
  scc_1ph_piline19 : simetranss/Lines/mate_1ph_piline  FF=60  conf=config 9  lenfeet=575  dmi=off  RR1=0.8  LL1=0.002  CC1=7e-9  lenkm=1
  scc_1ph_piline20 : simetranss/Lines/mate_1ph_piline  FF=60  conf=config 9  lenfeet=125  dmi=off  RR1=0.8  LL1=0.002  CC1=7e-9  lenkm=1
  scc_1ph_piline21 : simetranss/Lines/mate_1ph_piline  FF=60  conf=config 9  lenfeet=525  dmi=off  RR1=0.8  LL1=0.002  CC1=7e-9  lenkm=1
  scc_1ph_piline22 : simetranss/Lines/mate_1ph_piline  FF=60  conf=config 9  lenfeet=325  dmi=off  RR1=0.8  LL1=0.002  CC1=7e-9  lenkm=1
  scc_1ph_piline5 : simetranss/Lines/mate_1ph_piline  FF=60  conf=config 11  lenfeet=275  dmi=off  RR1=0.8  LL1=0.002  CC1=7e-9  lenkm=1
  scc_1ph_piline53 : simetranss/Lines/mate_1ph_piline  FF=60  conf=config 11  lenfeet=675  dmi=off  RR1=0.8  LL1=0.002  CC1=7e-9  lenkm=1
  scc_1ph_piline54 : simetranss/Lines/mate_1ph_piline  FF=60  conf=config 11  lenfeet=475  dmi=off  RR1=0.8  LL1=0.002  CC1=7e-9  lenkm=1
  scc_1ph_piline6 : simetranss/Lines/mate_1ph_piline  FF=60  conf=config 11  lenfeet=350  dmi=off  RR1=0.8  LL1=0.002  CC1=7e-9  lenkm=1
  scc_1ph_piline7 : simetranss/Lines/mate_1ph_piline  FF=60  conf=config 11  lenfeet=400  dmi=off  RR1=0.8  LL1=0.002  CC1=7e-9  lenkm=1
  scc_1ph_piline8 : simetranss/Lines/mate_1ph_piline  FF=60  conf=config 9  lenfeet=200  dmi=off  RR1=0.8  LL1=0.002  CC1=7e-9  lenkm=1
  scc_1ph_piline9 : simetranss/Lines/mate_1ph_piline  FF=60  conf=config 9  lenfeet=275  dmi=off  RR1=0.8  LL1=0.002  CC1=7e-9  lenkm=1
  scc_3ph_piline14 : simetranss/Lines/mate_3ph_piline  FF=60  conf=config 6  lenfeet=250  dmi=off  RR33=[1 0 0;0 1 0; 0 0 1]  LL33=[1 0 0;0 1 0; 0 0 1]  CC33=[1 0 0;0 1 0; 0 0 1]  lenkm=1
  scc_3ph_piline15 : simetranss/Lines/mate_3ph_piline  FF=60  conf=config 6  lenfeet=250  dmi=off  RR33=[1 0 0;0 1 0; 0 0 1]  LL33=[1 0 0;0 1 0; 0 0 1]  CC33=[1 0 0;0 1 0; 0 0 1]  lenkm=1
  scc_3ph_piline16 : simetranss/Lines/mate_3ph_piline  FF=60  conf=config 6  lenfeet=475  dmi=off  RR33=[1 0 0;0 1 0; 0 0 1]  LL33=[1 0 0;0 1 0; 0 0 1]  CC33=[1 0 0;0 1 0; 0 0 1]  lenkm=1
  scc_3ph_piline17 : simetranss/Lines/mate_3ph_piline  FF=60  conf=config 6  lenfeet=475  dmi=off  RR33=[1 0 0;0 1 0; 0 0 1]  LL33=[1 0 0;0 1 0; 0 0 1]  CC33=[1 0 0;0 1 0; 0 0 1]  lenkm=1
  scc_3ph_piline18 : simetranss/Lines/mate_3ph_piline  FF=60  conf=config 6  lenfeet=225  dmi=off  RR33=[1 0 0;0 1 0; 0 0 1]  LL33=[1 0 0;0 1 0; 0 0 1]  CC33=[1 0 0;0 1 0; 0 0 1]  lenkm=1
  scc_3ph_piline19 : simetranss/Lines/mate_3ph_piline  FF=60  conf=config 6  lenfeet=100  dmi=off  RR33=[1 0 0;0 1 0; 0 0 1]  LL33=[1 0 0;0 1 0; 0 0 1]  CC33=[1 0 0;0 1 0; 0 0 1]  lenkm=1
  scc_3ph_piline20 : simetranss/Lines/mate_3ph_piline  FF=60  conf=config 6  lenfeet=400  dmi=off  RR33=[1 0 0;0 1 0; 0 0 1]  LL33=[1 0 0;0 1 0; 0 0 1]  CC33=[1 0 0;0 1 0; 0 0 1]  lenkm=1
  scc_3ph_piline21 : simetranss/Lines/mate_3ph_piline  FF=60  conf=config 3  lenfeet=200  dmi=off  RR33=[1 0 0;0 1 0; 0 0 1]  LL33=[1 0 0;0 1 0; 0 0 1]  CC33=[1 0 0;0 1 0; 0 0 1]  lenkm=1
  scc_3ph_piline22 : simetranss/Lines/mate_3ph_piline  FF=60  conf=config 3  lenfeet=275  dmi=off  RR33=[1 0 0;0 1 0; 0 0 1]  LL33=[1 0 0;0 1 0; 0 0 1]  CC33=[1 0 0;0 1 0; 0 0 1]  lenkm=1
  scc_3ph_piline23 : simetranss/Lines/mate_3ph_piline  FF=60  conf=config 3  lenfeet=250  dmi=off  RR33=[1 0 0;0 1 0; 0 0 1]  LL33=[1 0 0;0 1 0; 0 0 1]  CC33=[1 0 0;0 1 0; 0 0 1]  lenkm=1
  scc_3ph_piline24 : simetranss/Lines/mate_3ph_piline  FF=60  conf=config 3  lenfeet=275  dmi=off  RR33=[1 0 0;0 1 0; 0 0 1]  LL33=[1 0 0;0 1 0; 0 0 1]  CC33=[1 0 0;0 1 0; 0 0 1]  lenkm=1
  scc_3ph_piline25 : simetranss/Lines/mate_3ph_piline  FF=60  conf=config 3  lenfeet=550  dmi=off  RR33=[1 0 0;0 1 0; 0 0 1]  LL33=[1 0 0;0 1 0; 0 0 1]  CC33=[1 0 0;0 1 0; 0 0 1]  lenkm=1
  scc_3ph_piline26 : simetranss/Lines/mate_3ph_piline  FF=60  conf=config 3  lenfeet=300  dmi=off  RR33=[1 0 0;0 1 0; 0 0 1]  LL33=[1 0 0;0 1 0; 0 0 1]  CC33=[1 0 0;0 1 0; 0 0 1]  lenkm=1
  scc_3ph_piline27 : simetranss/Lines/mate_3ph_piline  FF=60  conf=config 3  lenfeet=800  dmi=off  RR33=[1 0 0;0 1 0; 0 0 1]  LL33=[1 0 0;0 1 0; 0 0 1]  CC33=[1 0 0;0 1 0; 0 0 1]  lenkm=1
  scc_3ph_piline28 : simetranss/Lines/mate_3ph_piline  FF=60  conf=config 3  lenfeet=250  dmi=off  RR33=[1 0 0;0 1 0; 0 0 1]  LL33=[1 0 0;0 1 0; 0 0 1]  CC33=[1 0 0;0 1 0; 0 0 1]  lenkm=1
  scc_3ph_piline29 : simetranss/Lines/mate_3ph_piline  FF=60  conf=config 3  lenfeet=275  dmi=off  RR33=[1 0 0;0 1 0; 0 0 1]  LL33=[1 0 0;0 1 0; 0 0 1]  CC33=[1 0 0;0 1 0; 0 0 1]  lenkm=1
  scc_3ph_piline30 : simetranss/Lines/mate_3ph_piline  FF=60  conf=config 3  lenfeet=325  dmi=off  RR33=[1 0 0;0 1 0; 0 0 1]  LL33=[1 0 0;0 1 0; 0 0 1]  CC33=[1 0 0;0 1 0; 0 0 1]  lenkm=1
  scc_3ph_piline49 : simetranss/Lines/mate_3ph_piline  FF=60  conf=config 5  lenfeet=550  dmi=off  RR33=[1 0 0;0 1 0; 0 0 1]  LL33=[1 0 0;0 1 0; 0 0 1]  CC33=[1 0 0;0 1 0; 0 0 1]  lenkm=1
  scc_3ph_piline50 : simetranss/Lines/mate_3ph_piline  FF=60  conf=config 12  lenfeet=250  dmi=off  RR33=[1 0 0;0 1 0; 0 0 1]  LL33=[1 0 0;0 1 0; 0 0 1]  CC33=[1 0 0;0 1 0; 0 0 1]  lenkm=1
  scc_3ph_piline51 : simetranss/Lines/mate_3ph_piline  FF=60  conf=config 12  lenfeet=175  dmi=off  RR33=[1 0 0;0 1 0; 0 0 1]  LL33=[1 0 0;0 1 0; 0 0 1]  CC33=[1 0 0;0 1 0; 0 0 1]  lenkm=1
  scc_3ph_piline52 : simetranss/Lines/mate_3ph_piline  FF=60  conf=config 12  lenfeet=350  dmi=off  RR33=[1 0 0;0 1 0; 0 0 1]  LL33=[1 0 0;0 1 0; 0 0 1]  CC33=[1 0 0;0 1 0; 0 0 1]  lenkm=1
  scc_3ph_piline53 : simetranss/Lines/mate_3ph_piline  FF=60  conf=config 12  lenfeet=425  dmi=off  RR33=[1 0 0;0 1 0; 0 0 1]  LL33=[1 0 0;0 1 0; 0 0 1]  CC33=[1 0 0;0 1 0; 0 0 1]  lenkm=1
  scc_3ph_piline54 : simetranss/Lines/mate_3ph_piline  FF=60  conf=config 12  lenfeet=325  dmi=off  RR33=[1 0 0;0 1 0; 0 0 1]  LL33=[1 0 0;0 1 0; 0 0 1]  CC33=[1 0 0;0 1 0; 0 0 1]  lenkm=1
  scc_3ph_piline55 : simetranss/Lines/mate_3ph_piline  FF=60  conf=config 6  lenfeet=350  dmi=off  RR33=[1 0 0;0 1 0; 0 0 1]  LL33=[1 0 0;0 1 0; 0 0 1]  CC33=[1 0 0;0 1 0; 0 0 1]  lenkm=1
  sph10 : Subsystem
  sph11 : Subsystem
  sph12 : Subsystem
  sph13 : Subsystem
  sph14 : Subsystem
  sph15 : Subsystem
  sph16 : Subsystem
  sph17 : Subsystem
  sph18 : Subsystem
  sph19 : Subsystem
  sph20 : Subsystem
  sph45 : Subsystem
  sph46 : Subsystem
  sph47 : Subsystem
  sph48 : Subsystem
  sph49 : Subsystem
  sph50 : Subsystem
  sph52 : Subsystem
  sph9 : Subsystem
  ssc 3ph breaker1 : simetran/ssc 3ph breaker  Ron=1e-3  Roff=1e6
  ssc 3ph breaker5 : simetran/ssc 3ph breaker  Ron=1e-3  Roff=1e6
  abc : PMIOPort  Side=Right
  abc3 : PMIOPort  Port=2  Side=Left
  abc1 : PMIOPort  Port=3  Side=Left
  wires:
  cmd5/1 -> ssc 3ph breaker5/1
  cmd1/1 -> ssc 3ph breaker1/1
  connections:
  scc_3ph_piline53/RConn1 -- scc_3ph_piline54/RConn1 -- SPOT 65/LConn1
  scc_1ph_piline22/LConn1 -- SPOT 114/LConn1
  scc_3ph_piline17/RConn1 -- scc_3ph_piline19/RConn1 -- scc_3ph_piline18/LConn1
  scc_3ph_piline23/LConn1 -- 15/RConn1 -- sph14/LConn1 -- scc_3ph_piline55/LConn1
  sph47/RConn1 -- SPOT 64/LConn1
  scc_3ph_piline29/RConn1 -- 18/LConn1
  scc_3ph_piline49/RConn1 -- sph52/LConn1 -- scc_3ph_piline50/RConn1 -- 35/LConn1 -- ssc 3ph breaker5/LConn1
  scc_3ph_piline15/RConn1 -- 13/LConn1
  scc_3ph_piline25/RConn1 -- scc_3ph_piline26/LConn1 -- sph16/LConn1
  scc_3ph_piline14/LConn1 -- Solver Configuration1/RConn1 -- sph9/LConn1 -- scc_3ph_piline15/LConn1
  scc_1ph_piline6/LConn1 -- scc_1ph_piline7/RConn1 -- SPOT 74/LConn1
  scc_3ph_piline20/LConn1 -- scc_3ph_piline21/LConn1 -- abc1/RConn1 -- SimScape RL Load3/LConn1
  scc_3ph_piline52/RConn1 -- sph46/LConn1 -- scc_3ph_piline51/LConn1
  scc_3ph_piline20/RConn1 -- sph12/LConn1 -- scc_3ph_piline19/LConn1
  Two-Winding Transformer 4.16 kV/ 480V/RConn1 -- Resistance/LConn1
  scc_3ph_piline28/LConn1 -- ssc 3ph breaker1/LConn1
  sph10/RConn1 -- SPOT 83/LConn1
  18/RConn1 -- sph19/LConn1 -- scc_3ph_piline30/LConn1
  scc_3ph_piline49/LConn1 -- Two-Winding Transformer 4.16 kV/ 480V/LConn1
  SPOT 77/LConn1 -- sph12/RConn1
  16/RConn1 -- ssc 3ph breaker1/RConn1 -- scc_3ph_piline24/LConn1
  scc_1ph_piline54/RConn1 -- SPOT 85/LConn1
  SPOT 60/LConn1 -- sph52/RConn1
  scc_3ph_piline25/LConn1 -- sph15/LConn1 -- scc_3ph_piline24/RConn1
  13/RConn1 -- scc_3ph_piline16/LConn1 -- sph50/LConn1
  scc_1ph_piline19/LConn1 -- SPOT 111/LConn1
  SPOT 99/LConn1 -- sph16/RConn1
  20/RConn1 -- scc_1ph_piline20/RConn1 -- scc_1ph_piline19/RConn1
  scc_1ph_piline8/RConn1 -- sph14/RConn1
  sph48/RConn1 -- SPOT 62/LConn1
  scc_1ph_piline15/RConn1 -- sph19/RConn1
  sph13/RConn1 -- scc_1ph_piline5/RConn1
  scc_1ph_piline7/LConn1 -- SPOT 75/LConn1
  scc_1ph_piline13/LConn1 -- SPOT 103/LConn1 -- scc_1ph_piline14/RConn1
  scc_3ph_piline14/RConn1 -- MATE Unbalanced Load/LConn1 -- sph10/LConn1
  scc_1ph_piline16/LConn1 -- SPOT 107/LConn1
  36/RConn1 -- ssc 3ph breaker5/RConn1
  scc_1ph_piline14/LConn1 -- SPOT 104/LConn1
  scc_1ph_piline15/LConn1 -- scc_1ph_piline16/RConn1 -- SPOT 106/LConn1
  scc_3ph_piline22/LConn1 -- 14/RConn1
  20/LConn1 -- scc_1ph_piline18/LConn1
  scc_1ph_piline12/RConn1 -- sph18/RConn1
  scc_1ph_piline17/LConn1 -- scc_1ph_piline18/RConn1 -- SPOT 109/LConn1
  19/RConn1 -- abc/RConn1 -- sph20/LConn1
  SPOT 66/LConn1 -- sph45/RConn1
  19/LConn1 -- scc_3ph_piline30/RConn1
  scc_1ph_piline12/LConn1 -- scc_1ph_piline13/RConn1 -- SPOT 102/LConn1
  scc_3ph_piline52/LConn1 -- sph47/LConn1 -- scc_3ph_piline53/LConn1
  abc3/RConn1 -- 35/RConn1
  scc_1ph_piline11/LConn1 -- SPOT 71/LConn1
  sph46/RConn1 -- SPOT 63/LConn1
  scc_3ph_piline18/RConn1 -- sph49/LConn1
  36/LConn1 -- OLTC/LConn1
  SPOT 82/LConn1 -- sph9/RConn1
  scc_1ph_piline5/LConn1 -- scc_1ph_piline6/RConn1 -- SPOT 73/LConn1
  SPOT 100/LConn1 -- sph17/RConn1
  SPOT 80/LConn1 -- sph11/RConn1
  scc_1ph_piline8/LConn1 -- SPOT 68/LConn1 -- scc_1ph_piline9/RConn1
  scc_3ph_piline55/RConn1 -- OLTC/RConn1
  sph49/RConn1 -- SPOT 79/LConn1
  scc_3ph_piline16/RConn1 -- sph11/LConn1 -- scc_3ph_piline17/LConn1
  scc_1ph_piline10/LConn1 -- SPOT 70/LConn1 -- scc_1ph_piline11/RConn1
  scc_3ph_piline50/LConn1 -- sph48/LConn1 -- scc_3ph_piline51/RConn1
  scc_1ph_piline22/RConn1 -- SPOT 113/LConn1 -- scc_1ph_piline21/LConn1
  scc_1ph_piline53/RConn1 -- sph50/RConn1
  scc_1ph_piline20/LConn1 -- SPOT 112/LConn1 -- scc_1ph_piline21/RConn1
  scc_3ph_piline21/RConn1 -- sph13/LConn1 -- 14/LConn1
  scc_3ph_piline54/LConn1 -- sph45/LConn1
  scc_3ph_piline28/RConn1 -- 17/LConn1 -- sph18/LConn1
  scc_3ph_piline27/LConn1 -- sph17/LConn1 -- scc_3ph_piline26/RConn1
  17/RConn1 -- scc_3ph_piline29/LConn1
  scc_3ph_piline22/RConn1 -- 15/LConn1
  16/LConn1 -- scc_3ph_piline23/RConn1
  scc_1ph_piline10/RConn1 -- SPOT 69/LConn1 -- scc_1ph_piline9/LConn1
  scc_1ph_piline54/LConn1 -- SPOT 84/LConn1 -- scc_1ph_piline53/LConn1
  sph20/RConn1 -- scc_1ph_piline17/RConn1
  SPOT 98/LConn1 -- sph15/RConn1

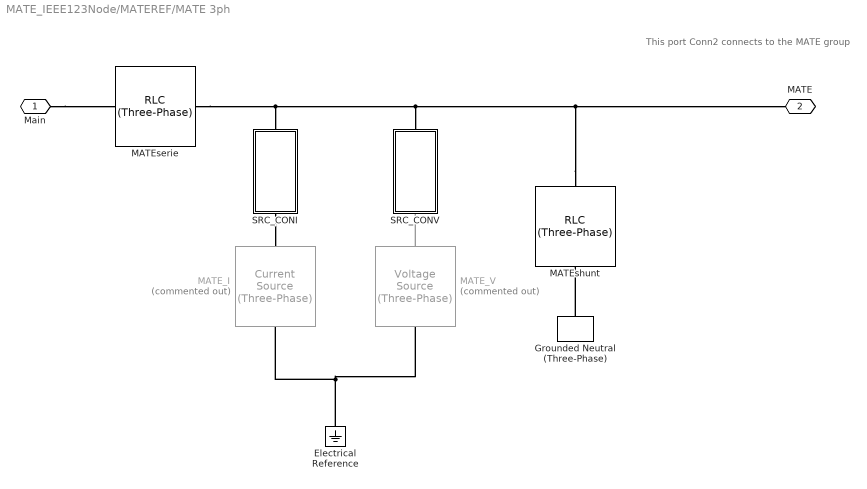
== system MATE_IEEE123Node/MATEREF/MATE 3ph ==
  note: This port Conn2 connects to the MATE group
  Electrical Reference : fl_lib/Electrical/Electrical Elements/Electrical Reference
  Grounded Neutral (Three-Phase) : ee_lib/Connectors & References/Grounded Neutral (Three-Phase)
  MATE_I : ee_lib/Sources/Current Source (Three-Phase)  Commented=on  iphase_rms=100 / sqrt(2) A  shift=0 deg  freq=60 Hz
      settings: InternalSimscapePortConfiguration="{\"Bottom\":[],\"Left\":[{\"id\":\"n\",\"label\":\"n\",\"type\":\"foundation.electrical.electrical\"}],\"Right\":[{\"id\":\"N\",\"label\":\"~\",\"type\":\"foundation.electrical.three_phase\"}],\"Top\":[]}"
  MATE_V : ee_lib/Sources/Voltage Source (Three-Phase)  Commented=on  vline_rms=0 V  shift=0 deg  freq=1 Hz  impedance_option=0  SShortCircuit=1e6 A*V  XR=15  R=0.0001 Ohm  L=3.97e-4 H  harmonic_option=0  harmonic_orders=[5, 7, 11, 13]  harmonic_ratios=[.1, .1, .1, .1]  G_parasitic=0 1/Ohm  I_specify=off  I_priority=None  I=[0, 0, 0] A  I_nominal_specify=off  I_nominal_value=1  I_nominal_unit=A
  MATEserie : ee_lib/Passive/RLC Assemblies/RLC (Three-Phase)  port_option=ee.enum.threePhasePort.composite  component_structure=ee.enum.rlc.structure.R  R=Rse Ohm  L=1e-3 H  C=1e-6 F  R_parasitic=0 Ohm  G_parasitic=0 1/Ohm  IL_specify=off  IL_priority=High  IL=[0, 0, 0] A  IL_nominal_specify=off  IL_nominal_value=1  IL_nominal_unit=A  VC_specify=off  VC_priority=High  VC=[0, 0, 0] V  VC_nominal_specify=off  VC_nominal_value=1  VC_nominal_unit=V
      settings: InternalSimscapePortConfiguration="{\"Bottom\":[],\"Left\":[{\"id\":\"N1\",\"label\":\"~1\",\"type\":\"foundation.electrical.three_phase\"}],\"Right\":[{\"id\":\"N2\",\"label\":\"~2\",\"type\":\"foundation.electrical.three_phase\"}],\"Top\":[]}"
  MATEshunt : ee_lib/Passive/RLC Assemblies/RLC (Three-Phase)  port_option=ee.enum.threePhasePort.composite  component_structure=ee.enum.rlc.structure.R  R=Rsh Ohm  L=1e-3 H  C=1e-6 F  R_parasitic=0 Ohm  G_parasitic=0 1/Ohm  IL_specify=off  IL_priority=High  IL=[0, 0, 0] A  IL_nominal_specify=off  IL_nominal_value=1  IL_nominal_unit=A  VC_specify=off  VC_priority=High  VC=[0, 0, 0] V  VC_nominal_specify=off  VC_nominal_value=1  VC_nominal_unit=V
      settings: InternalSimscapePortConfiguration="{\"Bottom\":[],\"Left\":[{\"id\":\"N1\",\"label\":\"~1\",\"type\":\"foundation.electrical.three_phase\"}],\"Right\":[{\"id\":\"N2\",\"label\":\"~2\",\"type\":\"foundation.electrical.three_phase\"}],\"Top\":[]}"
  SRC_CONI : Subsystem
  SRC_CONV : Subsystem
  Main : PMIOPort  Side=Left
  MATE : PMIOPort  Port=2  Side=Right
  connections:
  Main/RConn1 -- MATEserie/LConn1
  Grounded Neutral (Three-Phase)/LConn1 -- MATEshunt/LConn1
  SRC_CONI/RConn1 -- MATE_I/RConn1
  MATE_V/RConn1 -- SRC_CONV/RConn1
  MATE_V/LConn1 -- MATE_I/LConn1 -- Electrical Reference/LConn1
  MATEshunt/RConn1 -- MATE/RConn1 -- SRC_CONV/LConn1 -- MATEserie/RConn1 -- SRC_CONI/LConn1

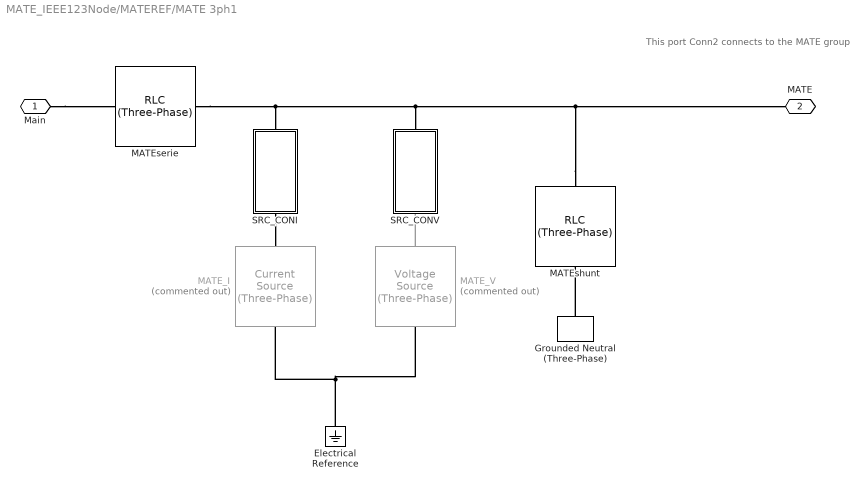
== system MATE_IEEE123Node/MATEREF/MATE 3ph1 ==
  note: This port Conn2 connects to the MATE group
  Electrical Reference : fl_lib/Electrical/Electrical Elements/Electrical Reference
  Grounded Neutral (Three-Phase) : ee_lib/Connectors & References/Grounded Neutral (Three-Phase)
  MATE_I : ee_lib/Sources/Current Source (Three-Phase)  Commented=on  iphase_rms=100 / sqrt(2) A  shift=0 deg  freq=60 Hz
      settings: InternalSimscapePortConfiguration="{\"Bottom\":[],\"Left\":[{\"id\":\"n\",\"label\":\"n\",\"type\":\"foundation.electrical.electrical\"}],\"Right\":[{\"id\":\"N\",\"label\":\"~\",\"type\":\"foundation.electrical.three_phase\"}],\"Top\":[]}"
  MATE_V : ee_lib/Sources/Voltage Source (Three-Phase)  Commented=on  vline_rms=0 V  shift=0 deg  freq=1 Hz  impedance_option=0  SShortCircuit=1e6 A*V  XR=15  R=0.0001 Ohm  L=3.97e-4 H  harmonic_option=0  harmonic_orders=[5, 7, 11, 13]  harmonic_ratios=[.1, .1, .1, .1]  G_parasitic=0 1/Ohm  I_specify=off  I_priority=None  I=[0, 0, 0] A  I_nominal_specify=off  I_nominal_value=1  I_nominal_unit=A
  MATEserie : ee_lib/Passive/RLC Assemblies/RLC (Three-Phase)  port_option=ee.enum.threePhasePort.composite  component_structure=ee.enum.rlc.structure.R  R=Rse Ohm  L=1e-3 H  C=1e-6 F  R_parasitic=0 Ohm  G_parasitic=0 1/Ohm  IL_specify=off  IL_priority=High  IL=[0, 0, 0] A  IL_nominal_specify=off  IL_nominal_value=1  IL_nominal_unit=A  VC_specify=off  VC_priority=High  VC=[0, 0, 0] V  VC_nominal_specify=off  VC_nominal_value=1  VC_nominal_unit=V
      settings: InternalSimscapePortConfiguration="{\"Bottom\":[],\"Left\":[{\"id\":\"N1\",\"label\":\"~1\",\"type\":\"foundation.electrical.three_phase\"}],\"Right\":[{\"id\":\"N2\",\"label\":\"~2\",\"type\":\"foundation.electrical.three_phase\"}],\"Top\":[]}"
  MATEshunt : ee_lib/Passive/RLC Assemblies/RLC (Three-Phase)  port_option=ee.enum.threePhasePort.composite  component_structure=ee.enum.rlc.structure.R  R=Rsh Ohm  L=1e-3 H  C=1e-6 F  R_parasitic=0 Ohm  G_parasitic=0 1/Ohm  IL_specify=off  IL_priority=High  IL=[0, 0, 0] A  IL_nominal_specify=off  IL_nominal_value=1  IL_nominal_unit=A  VC_specify=off  VC_priority=High  VC=[0, 0, 0] V  VC_nominal_specify=off  VC_nominal_value=1  VC_nominal_unit=V
      settings: InternalSimscapePortConfiguration="{\"Bottom\":[],\"Left\":[{\"id\":\"N1\",\"label\":\"~1\",\"type\":\"foundation.electrical.three_phase\"}],\"Right\":[{\"id\":\"N2\",\"label\":\"~2\",\"type\":\"foundation.electrical.three_phase\"}],\"Top\":[]}"
  SRC_CONI : Subsystem
  SRC_CONV : Subsystem
  Main : PMIOPort  Side=Left
  MATE : PMIOPort  Port=2  Side=Right
  connections:
  Main/RConn1 -- MATEserie/LConn1
  Grounded Neutral (Three-Phase)/LConn1 -- MATEshunt/LConn1
  SRC_CONI/RConn1 -- MATE_I/RConn1
  MATE_V/RConn1 -- SRC_CONV/RConn1
  MATE_V/LConn1 -- MATE_I/LConn1 -- Electrical Reference/LConn1
  MATEshunt/RConn1 -- MATE/RConn1 -- SRC_CONV/LConn1 -- MATEserie/RConn1 -- SRC_CONI/LConn1
